simulink library "optimizeAltitude_ul"  (R2022a)
settings: Solver=VariableStepAuto  StartTime=0.0  StopTime=10.0  RelTol=1e-3
values from neighbouring files (symbols this model uses):
  hiLvlCtrl = block.DialogPrm(2).Data    [optimizeAltitude_Lvl2SFun.m]    (also in optimizeThrLenghtAndElevation_Lvl2sFun.m; optimizeTrajectory_Lvl2SFun.m)
  mpckfgp = block.DialogPrm(1).Data    [optimizeAltitude_Lvl2SFun.m]    (also in optimizeAltitude_init.m = GP.KalmanFilteredGaussianProcess(hiLvlCtrl.spatialCovFn,    ; optimizeTrajectory_Lvl2SFun.m; optimizeTrajectory_init.m = GP.KalmanFilteredGaussianProcess(hiLvlCtrl.spatialCovFn,    )
settings Model: Creator=Ayaz  LastModifiedBy=lhill8
settings SolverCC: AlgebraicLoopSolver=TrustRegion
settings DebuggingCC: UnconnectedInputMsg=warning  UnconnectedOutputMsg=warning  UnconnectedLineMsg=warning  SFMachineParentedDataDiag=warning

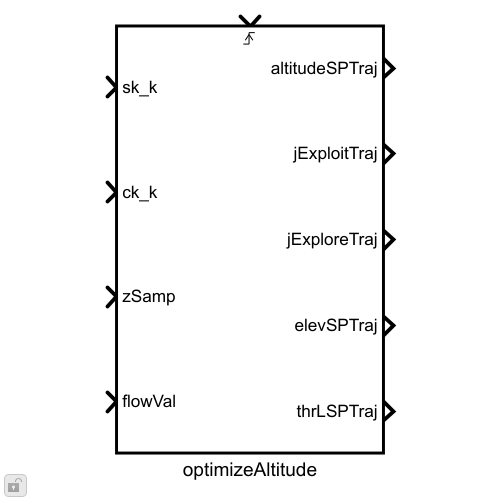
[thumbnail: Simulink's stored preview of the top-level diagram]
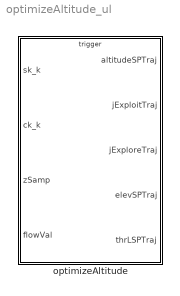
== system optimizeAltitude_ul ==
  optimizeAltitude : Subsystem  mask{hiLvlCtrl=hiLvlCtrl}
      mask prompts: hiLvlCtrl "High level controller object"
      mask init:
      | optimizeAltitude_init

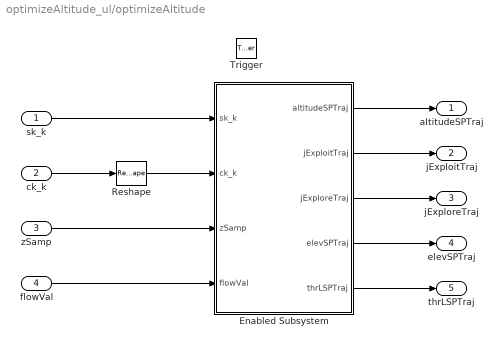
== system optimizeAltitude_ul/optimizeAltitude ==
  sk_k : Inport
  ck_k : Inport  Port=2
  zSamp : Inport  Port=3
  flowVal : Inport  Port=4
  Trigger : TriggerPort  VariantControl=Variant
  Enabled Subsystem : Subsystem  TreatAsAtomicUnit=on
  Reshape : Reshape  OutputDimensionality=Column vector (2-D)
  altitudeSPTraj : Outport
  jExploitTraj : Outport  Port=2
  jExploreTraj : Outport  Port=3
  elevSPTraj : Outport  Port=4
  thrLSPTraj : Outport  Port=5
  wires:
  flowVal/1 -> Enabled Subsystem/4(flowVal)
  zSamp/1 -> Enabled Subsystem/3(zSamp)
  ck_k/1 -> Reshape/1
  sk_k/1 -> Enabled Subsystem/1(sk_k)
  Reshape/1 -> Enabled Subsystem/2(ck_k)
  Enabled Subsystem/5(thrLSPTraj) -> thrLSPTraj/1
  Enabled Subsystem/1(altitudeSPTraj) -> altitudeSPTraj/1
  Enabled Subsystem/2(jExploitTraj) -> jExploitTraj/1
  Enabled Subsystem/3(jExploreTraj) -> jExploreTraj/1
  Enabled Subsystem/4(elevSPTraj) -> elevSPTraj/1

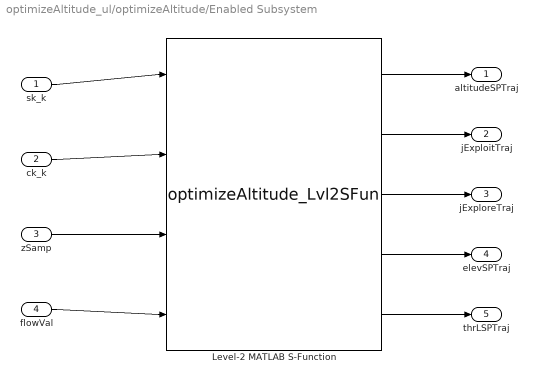
== system optimizeAltitude_ul/optimizeAltitude/Enabled Subsystem ==
  sk_k : Inport
  ck_k : Inport  Port=2
  zSamp : Inport  Port=3
  flowVal : Inport  Port=4
  Level-2 MATLAB S-Function : M-S-Function  FunctionName=optimizeAltitude_Lvl2SFun  Parameters=mpckfgp,hiLvlCtrl
  altitudeSPTraj : Outport
  jExploitTraj : Outport  Port=2
  jExploreTraj : Outport  Port=3
  elevSPTraj : Outport  Port=4
  thrLSPTraj : Outport  Port=5
  wires:
  Level-2 MATLAB S-Function/1 -> altitudeSPTraj/1
  Level-2 MATLAB S-Function/2 -> jExploitTraj/1
  Level-2 MATLAB S-Function/3 -> jExploreTraj/1
  flowVal/1 -> Level-2 MATLAB S-Function/4
  zSamp/1 -> Level-2 MATLAB S-Function/3
  sk_k/1 -> Level-2 MATLAB S-Function/1
  ck_k/1 -> Level-2 MATLAB S-Function/2
  Level-2 MATLAB S-Function/5 -> thrLSPTraj/1
  Level-2 MATLAB S-Function/4 -> elevSPTraj/1
